simulink model "arm"  (R2018b)
settings: Solver=ode4  StartTime=0  StopTime=10  FixedStep=0.0005  RelTol=1e-7  AbsTol=1e-9  EnableMultiTasking=on
settings Model: Creator=Laksh  LastModifiedBy=visak
settings SolverCC: AutoScaleAbsTol=off  MaxConsecutiveMinStep=10  AlgebraicLoopSolver=LineSearch
settings DataIOCC: SaveFormat=StructureWithTime  SignalLogging=off  ReturnWorkspaceOutputs=on
settings OptimizationCC: LifeSpan=inf
settings DebuggingCC: ReadBeforeWriteMsg=DisableAll  WriteAfterWriteMsg=DisableAll  WriteAfterReadMsg=DisableAll  AlgebraicLoopMsg=none  MultiTaskDSMMsg=none  LibraryContextMissingDiagnostic=none  SFUnexpectedBacktrackingDiag=warning  SFNoUnconditionalDefaultTransitionDiag=warning  SFExecutionAtInitializationDiag=none
settings ModelReferenceCC: UpdateModelReferenceTargets=IfOutOfDate  ModelReferenceMinAlgLoopOccurrences=on
settings SFSimCC: SFSimEcho=off  SimUseLocalCustomCode=off
settings RTWCC: RTWUseLocalCustomCode=off
settings CodeAppCC: StateflowObjectComments=on
settings GRTTargetCC: TargetLangStandard=C89/C90 (ANSI)  GeneratePreprocessorConditionals=Disable all
settings ConfigComp: CovMetricSettings=dw  CovHtmlReporting=on  CovSaveCumulativeToWorkspaceVar=on  CovSaveSingleToWorkspaceVar=on  CovExternalEMLEnable=off

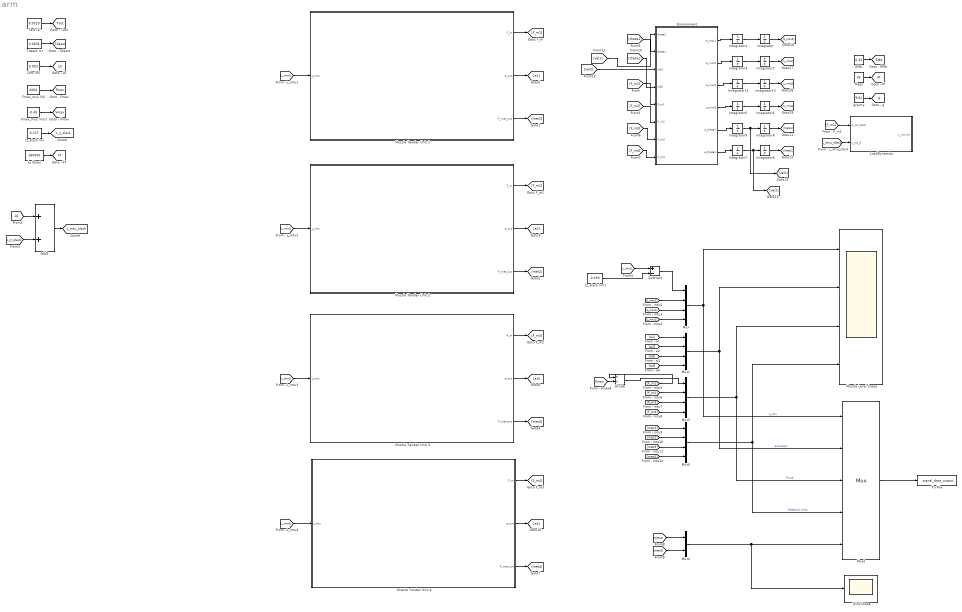
== system arm ==
  Add1 : Sum
  Divide : Product  Inputs=*/
  EMA : Constant  Value=0.33
  Environment : MATLAB Function  TreatAsAtomicUnit=on
  Fmax_mus (N) : Constant  Value=6000
  Integrator : Integrator  InitialCondition=0.05
  Integrator{1..11} (11 alike) : Integrator
  Joint Scope : Scope
  L0m (m) : Constant  Value=0.055
  LoadDynamics : Subsystem
  Lt_slack (m) : Constant  Value=0.237
  Lt_slack (m)1 : Constant  Value=0.293
  Mass : Constant  Value=35
  Muscle Level Scope : Scope  NumInputPorts=4
  Muscle Tenden Unit 1 : Subsystem
  Muscle Tenden Unit 2 : Subsystem
  Muscle Tenden Unit 3 : Subsystem
  Muscle Tenden Unit 4 : Subsystem
  Mux{,1,3,5} (4 alike) : Mux
  Mux2 : Mux  Inputs=5
      settings: DisplayOption=signals
  Mux4 : Mux  Inputs=2
  Subtract : Sum  Inputs=+-
  Tact (s) : Constant  Value=0.0329  VectorParams1D=off
  Tdeact (s) : Constant  Value=0.0905
  To File : ToFile  Filename=signal_data_output  MatrixName=data  SaveFormat=Timeseries
  Vmax_mus (m\s) : Constant  Value=-0.45
  gravity : Constant  Value=9.81
  kt (N\m) : Constant  Value=180000
  tag scope: EMA=global, Fmax=global, L0=global, L_mtu_slack=global, L_t_slack=global, M=global, Tact=global, Tdeact=global, Vmax=global, g=global, kT=global
  wires:
  Mux2/1 -> To File/1
  Tact (s)/1 -> [Tact]
  Tdeact (s)/1 -> [Tdeact]
  L0m (m)/1 -> [L0]
  Fmax_mus (N)/1 -> [Fmax]
  Vmax_mus (m\s)/1 -> [Vmax]
  Lt_slack (m)/1 -> [L_t_slack]
  [L_t_slack] -> Add1/2
  Add1/1 -> [L_mtu_slack]
  [L0] -> Add1/1
  kt (N\m)/1 -> [kT]
  [a1] -> Mux1/1
  [a2] -> Mux1/2
  Mux1/1 -> Muscle Level Scope/2, Mux2/2  "activation"
  Muscle Tenden Unit 1/1(F_m) -> [F_m1]
  [L_mtu1] -> Muscle Tenden Unit 1/1("L_mtu ")
  Muscle Tenden Unit 1/2(a_out) -> [a1]
  [F_m1] -> Environment/5(F_m1)
  [F_m2] -> Environment/6(F_m2)
  [F_m3] -> Environment/7(F_m3)
  [F_m4] -> Environment/8(F_m4)
  Environment/2(a_mtu2) -> Integrator3/1
  Muscle Tenden Unit 1/3(P_met_out) -> [met1]
  Muscle Tenden Unit 2/2(a_out) -> [a2]
  [L_mtu2] -> Muscle Tenden Unit 2/1("L_mtu ")
  Muscle Tenden Unit 2/1(F_m) -> [F_m2]
  Muscle Tenden Unit 2/3(P_met_out) -> [met2]
  Muscle Tenden Unit 3/3(P_met_out) -> [met3]
  Muscle Tenden Unit 3/1(F_m) -> [F_m3]
  [L_mtu3] -> Muscle Tenden Unit 3/1("L_mtu ")
  Muscle Tenden Unit 3/2(a_out) -> [a3]
  Muscle Tenden Unit 4/2(a_out) -> [a4]
  [L_mtu4] -> Muscle Tenden Unit 4/1("L_mtu ")
  Muscle Tenden Unit 4/1(F_m) -> [F_m4]
  Muscle Tenden Unit 4/3(P_met_out) -> [met4]
  [theta1] -> Mux4/1
  [theta2] -> Mux4/2
  [a3] -> Mux1/3
  [a4] -> Mux1/4
  [L_mtu1] -> Mux/3
  [L_mtu1] -> Mux/2
  [L_mtu1] -> Mux/4
  [F_m4] -> Mux3/4
  [F_m1] -> Divide/1
  [F_m3] -> Mux3/3
  [F_m2] -> Mux3/2
  Mux3/1 -> Muscle Level Scope/3, Mux2/3  "Force"
  Mux4/1 -> Mux2/5, Joint Scope/1
  Mux5/1 -> Muscle Level Scope/4, Mux2/4  "Metabolic Cost"
  [met2] -> Mux5/2
  [met3] -> Mux5/3
  [met1] -> Mux5/1
  [met4] -> Mux5/4
  Mux/1 -> Mux2/1, Muscle Level Scope/1  "L_mtu"
  Environment/1(a_mtu1) -> Integrator1/1
  Integrator1/1 -> Integrator/1
  Integrator3/1 -> Integrator2/1
  Integrator2/1 -> [L_mtu2]
  Integrator5/1 -> Integrator4/1
  Environment/4(a_mtu4) -> Integrator5/1
  Environment/6(a_theta2) -> Integrator7/1
  Integrator7/1 -> [vel2], Integrator6/1
  Integrator6/1 -> [theta2]
  Integrator4/1 -> [L_mtu4]
  Integrator8/1 -> [theta1]
  Integrator9/1 -> [vel1], Integrator8/1
  Environment/5(a_theta1) -> Integrator9/1
  Integrator11/1 -> Integrator10/1
  Environment/3(a_mtu3) -> Integrator11/1
  Integrator10/1 -> [L_mtu3]
  Integrator/1 -> [L_mtu1]
  [Fmax] -> Divide/2
  Divide/1 -> Mux3/1
  [L_mtu_slack] -> LoadDynamics/2(L_mt_0)
  [F_m1] -> LoadDynamics/1(F_mt_total)
  Mass/1 -> [M]
  gravity/1 -> [g]
  EMA/1 -> [EMA]
  Lt_slack (m)1/1 -> Subtract/2
  Subtract/1 -> Mux/1
  [L_mtu1] -> Subtract/1
  [theta2] -> Environment/3(vel1)
  [vel2] -> Environment/4(vel2)
  [vel1] -> Environment/1(theta2)
  [theta1] -> Environment/2(theta1)

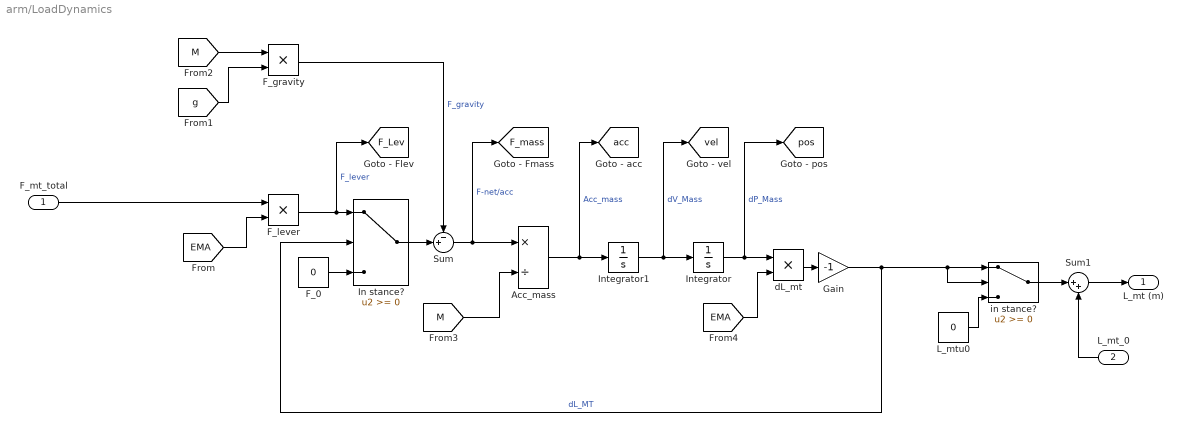
== system arm/LoadDynamics ==
  F_mt_total : Inport
  L_mt_0 : Inport  Port=2
  Acc_mass : Product  Inputs=*/
  F_0 : Constant  Value=0
  F_gravity : Product  RndMeth=Zero
  F_lever : Product  RndMeth=Zero
  Gain : Gain  Gain=-1
  In stance? : Switch
  Integrator : Integrator  InitialCondition=0.05
  Integrator1 : Integrator
  L_mtu0 : Constant  Value=0
  Sum : Sum  Inputs=-+|
  Sum1 : Sum  Inputs=|++
  dL_mt : Product  RndMeth=Zero
  "in stance? " : Switch
  L_mt (m) : Outport
  tag scope: F_Lev=global, F_mass=global, acc=global, pos=global, vel=global
  wires:
  Integrator1/1 -> [vel], Integrator/1  "dV_Mass"
  Sum1/1 -> L_mt (m)/1
  L_mt_0/1 -> Sum1/2
  Acc_mass/1 -> [acc], Integrator1/1  "Acc_mass"
  Sum/1 -> [F_mass], Acc_mass/1  "F-net/acc"
  F_mt_total/1 -> F_lever/1
  Gain/1 -> "in stance? "/2, "in stance? "/1, In stance?/2  "dL_MT"
  dL_mt/1 -> Gain/1
  F_lever/1 -> [F_Lev], In stance?/1  "F_lever"
  L_mtu0/1 -> "in stance? "/3
  "in stance? "/1 -> Sum1/1
  [M] -> F_gravity/1
  [g] -> F_gravity/2
  [EMA] -> F_lever/2
  F_0/1 -> In stance?/3
  Integrator/1 -> [pos], dL_mt/1  "dP_Mass"
  [M] -> Acc_mass/2
  In stance?/1 -> Sum/2
  F_gravity/1 -> Sum/1  "F_gravity"
  [EMA] -> dL_mt/2

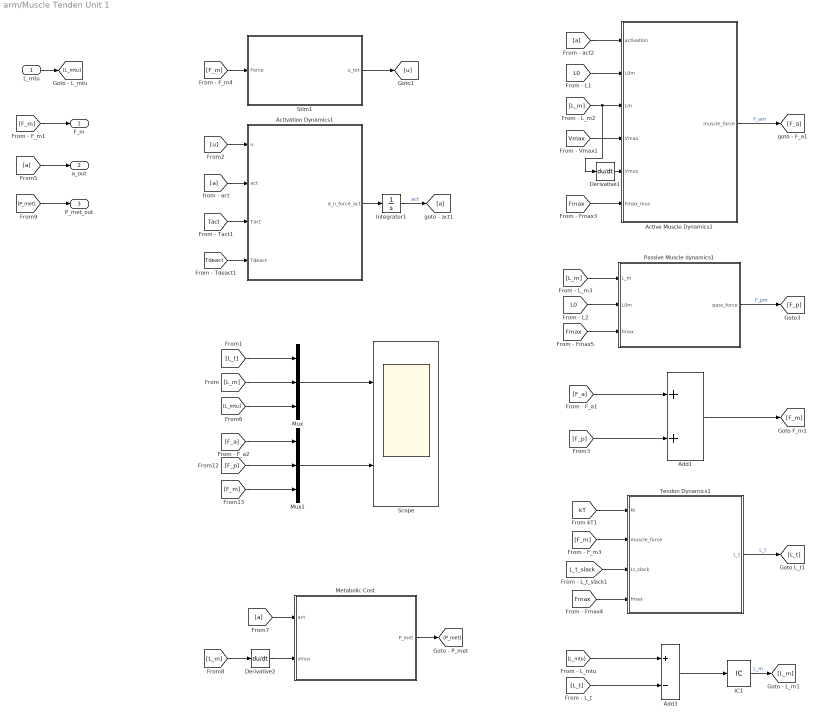
== system arm/Muscle Tenden Unit 1 ==
  "L_mtu " : Inport
  Activation Dynamics1 : MATLAB Function  TreatAsAtomicUnit=on
  Active Muscle Dynamics1 : MATLAB Function
  Add1 : Sum
  Add3 : Sum  Inputs=+-
  Derivative1 : Derivative
  Derivative2 : Derivative
  IC1 : InitialCondition  Value=0.05
  Integrator1 : Integrator
  Metabolic Cost : MATLAB Function
  Mux : Mux  Inputs=3
  Mux1 : Mux  Inputs=3
  Passive Muscle dynamics1 : MATLAB Function
  Scope : Scope  NumInputPorts=2
  Stim1 : Subsystem
  Tendon Dynamics1 : MATLAB Function
  F_m : Outport
  a_out : Outport  Port=2
  P_met_out : Outport  Port=3
  wires:
  [F_m] -> F_m/1
  Activation Dynamics1/1(d_n_force_act) -> Integrator1/1
  [F_p] -> Add1/2
  [L_m] -> Passive Muscle dynamics1/1(L_m)
  [L_mtu] -> Add3/1
  [L_m] -> Derivative1/1, Active Muscle Dynamics1/3(Lm)
  Stim1/1(u_tot) -> [u]
  [F_m] -> Stim1/1(Force)
  Tendon Dynamics1/1(L_t) -> [L_t]  "L_t"
  Add1/1 -> [F_m]
  [a] -> Active Muscle Dynamics1/1(activation)
  Passive Muscle dynamics1/1(pass_force) -> [F_p]  "F_pm"
  [Fmax] -> Passive Muscle dynamics1/3(fmax)
  [kT] -> Tendon Dynamics1/1(kt)
  [L_t] -> Add3/2
  [Vmax] -> Active Muscle Dynamics1/4(Vmax)
  [Fmax] -> Tendon Dynamics1/4(fmax)
  [L0] -> Passive Muscle dynamics1/2(L0m)
  [L_t_slack] -> Tendon Dynamics1/3(Lt_slack)
  [Fmax] -> Active Muscle Dynamics1/6(Fmax_mus)
  [Tact] -> Activation Dynamics1/3(Tact)
  [L0] -> Active Muscle Dynamics1/2(L0m)
  IC1/1 -> [L_m]  "L_m"
  [u] -> Activation Dynamics1/1(u)
  Integrator1/1 -> [a]  "act"
  [F_a] -> Add1/1
  [Tdeact] -> Activation Dynamics1/4(Tdeact)
  Derivative1/1 -> Active Muscle Dynamics1/5(Vmus)
  [a] -> Activation Dynamics1/2(act)
  [F_m] -> Tendon Dynamics1/2(muscle_force)
  Active Muscle Dynamics1/1(muscle_force) -> [F_a]  "F_am"
  Add3/1 -> IC1/1
  "L_mtu "/1 -> [L_mtu]
  [L_m] -> Mux/2
  [L_t] -> Mux/1
  [a] -> a_out/1
  [a] -> Metabolic Cost/1(act)
  [L_m] -> Derivative2/1
  Derivative2/1 -> Metabolic Cost/2(vmus)
  Metabolic Cost/1(P_met) -> [P_met]
  [P_met] -> P_met_out/1
  [L_mtu] -> Mux/3
  Mux/1 -> Scope/1
  [F_a] -> Mux1/1
  [F_m] -> Mux1/3
  [F_p] -> Mux1/2
  Mux1/1 -> Scope/2

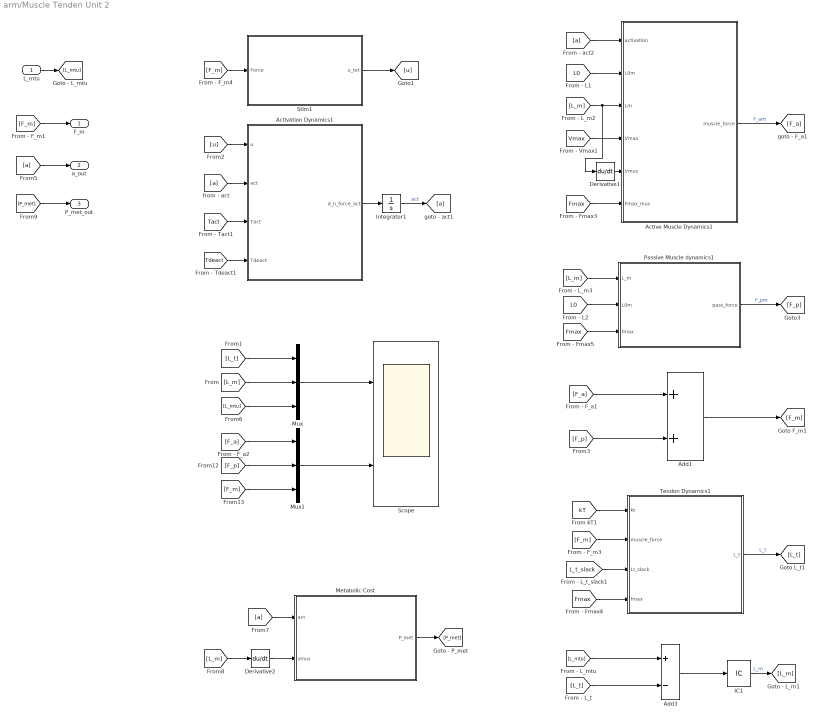
== system arm/Muscle Tenden Unit 2 ==
  "L_mtu " : Inport
  Activation Dynamics1 : MATLAB Function  TreatAsAtomicUnit=on
  Active Muscle Dynamics1 : MATLAB Function
  Add1 : Sum
  Add3 : Sum  Inputs=+-
  Derivative1 : Derivative
  Derivative2 : Derivative
  IC1 : InitialCondition  Value=0.05
  Integrator1 : Integrator
  Metabolic Cost : MATLAB Function
  Mux : Mux  Inputs=3
  Mux1 : Mux  Inputs=3
  Passive Muscle dynamics1 : MATLAB Function
  Scope : Scope  NumInputPorts=2
  Stim1 : Subsystem
  Tendon Dynamics1 : MATLAB Function
  F_m : Outport
  a_out : Outport  Port=2
  P_met_out : Outport  Port=3
  wires:
  [F_m] -> F_m/1
  Activation Dynamics1/1(d_n_force_act) -> Integrator1/1
  [F_p] -> Add1/2
  [L_m] -> Passive Muscle dynamics1/1(L_m)
  [L_mtu] -> Add3/1
  [L_m] -> Derivative1/1, Active Muscle Dynamics1/3(Lm)
  Stim1/1(u_tot) -> [u]
  [F_m] -> Stim1/1(Force)
  Tendon Dynamics1/1(L_t) -> [L_t]  "L_t"
  Add1/1 -> [F_m]
  [a] -> Active Muscle Dynamics1/1(activation)
  Passive Muscle dynamics1/1(pass_force) -> [F_p]  "F_pm"
  [Fmax] -> Passive Muscle dynamics1/3(fmax)
  [kT] -> Tendon Dynamics1/1(kt)
  [L_t] -> Add3/2
  [Vmax] -> Active Muscle Dynamics1/4(Vmax)
  [Fmax] -> Tendon Dynamics1/4(fmax)
  [L0] -> Passive Muscle dynamics1/2(L0m)
  [L_t_slack] -> Tendon Dynamics1/3(Lt_slack)
  [Fmax] -> Active Muscle Dynamics1/6(Fmax_mus)
  [Tact] -> Activation Dynamics1/3(Tact)
  [L0] -> Active Muscle Dynamics1/2(L0m)
  IC1/1 -> [L_m]  "L_m"
  [u] -> Activation Dynamics1/1(u)
  Integrator1/1 -> [a]  "act"
  [F_a] -> Add1/1
  [Tdeact] -> Activation Dynamics1/4(Tdeact)
  Derivative1/1 -> Active Muscle Dynamics1/5(Vmus)
  [a] -> Activation Dynamics1/2(act)
  [F_m] -> Tendon Dynamics1/2(muscle_force)
  Active Muscle Dynamics1/1(muscle_force) -> [F_a]  "F_am"
  Add3/1 -> IC1/1
  "L_mtu "/1 -> [L_mtu]
  [L_m] -> Mux/2
  [L_t] -> Mux/1
  [a] -> a_out/1
  [a] -> Metabolic Cost/1(act)
  [L_m] -> Derivative2/1
  Derivative2/1 -> Metabolic Cost/2(vmus)
  Metabolic Cost/1(P_met) -> [P_met]
  [P_met] -> P_met_out/1
  [L_mtu] -> Mux/3
  Mux/1 -> Scope/1
  [F_a] -> Mux1/1
  [F_m] -> Mux1/3
  [F_p] -> Mux1/2
  Mux1/1 -> Scope/2

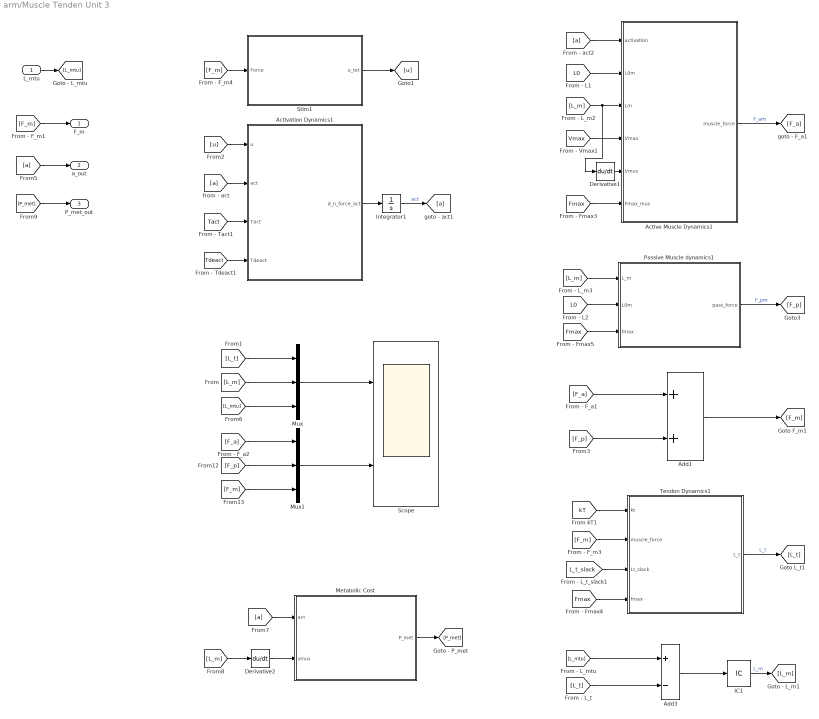
== system arm/Muscle Tenden Unit 3 ==
  "L_mtu " : Inport
  Activation Dynamics1 : MATLAB Function  TreatAsAtomicUnit=on
  Active Muscle Dynamics1 : MATLAB Function
  Add1 : Sum
  Add3 : Sum  Inputs=+-
  Derivative1 : Derivative
  Derivative2 : Derivative
  IC1 : InitialCondition  Value=0.05
  Integrator1 : Integrator
  Metabolic Cost : MATLAB Function
  Mux : Mux  Inputs=3
  Mux1 : Mux  Inputs=3
  Passive Muscle dynamics1 : MATLAB Function
  Scope : Scope  NumInputPorts=2
  Stim1 : Subsystem
  Tendon Dynamics1 : MATLAB Function
  F_m : Outport
  a_out : Outport  Port=2
  P_met_out : Outport  Port=3
  wires:
  [F_m] -> F_m/1
  Activation Dynamics1/1(d_n_force_act) -> Integrator1/1
  [F_p] -> Add1/2
  [L_m] -> Passive Muscle dynamics1/1(L_m)
  [L_mtu] -> Add3/1
  [L_m] -> Derivative1/1, Active Muscle Dynamics1/3(Lm)
  Stim1/1(u_tot) -> [u]
  [F_m] -> Stim1/1(Force)
  Tendon Dynamics1/1(L_t) -> [L_t]  "L_t"
  Add1/1 -> [F_m]
  [a] -> Active Muscle Dynamics1/1(activation)
  Passive Muscle dynamics1/1(pass_force) -> [F_p]  "F_pm"
  [Fmax] -> Passive Muscle dynamics1/3(fmax)
  [kT] -> Tendon Dynamics1/1(kt)
  [L_t] -> Add3/2
  [Vmax] -> Active Muscle Dynamics1/4(Vmax)
  [Fmax] -> Tendon Dynamics1/4(fmax)
  [L0] -> Passive Muscle dynamics1/2(L0m)
  [L_t_slack] -> Tendon Dynamics1/3(Lt_slack)
  [Fmax] -> Active Muscle Dynamics1/6(Fmax_mus)
  [Tact] -> Activation Dynamics1/3(Tact)
  [L0] -> Active Muscle Dynamics1/2(L0m)
  IC1/1 -> [L_m]  "L_m"
  [u] -> Activation Dynamics1/1(u)
  Integrator1/1 -> [a]  "act"
  [F_a] -> Add1/1
  [Tdeact] -> Activation Dynamics1/4(Tdeact)
  Derivative1/1 -> Active Muscle Dynamics1/5(Vmus)
  [a] -> Activation Dynamics1/2(act)
  [F_m] -> Tendon Dynamics1/2(muscle_force)
  Active Muscle Dynamics1/1(muscle_force) -> [F_a]  "F_am"
  Add3/1 -> IC1/1
  "L_mtu "/1 -> [L_mtu]
  [L_m] -> Mux/2
  [L_t] -> Mux/1
  [a] -> a_out/1
  [a] -> Metabolic Cost/1(act)
  [L_m] -> Derivative2/1
  Derivative2/1 -> Metabolic Cost/2(vmus)
  Metabolic Cost/1(P_met) -> [P_met]
  [P_met] -> P_met_out/1
  [L_mtu] -> Mux/3
  Mux/1 -> Scope/1
  [F_a] -> Mux1/1
  [F_m] -> Mux1/3
  [F_p] -> Mux1/2
  Mux1/1 -> Scope/2

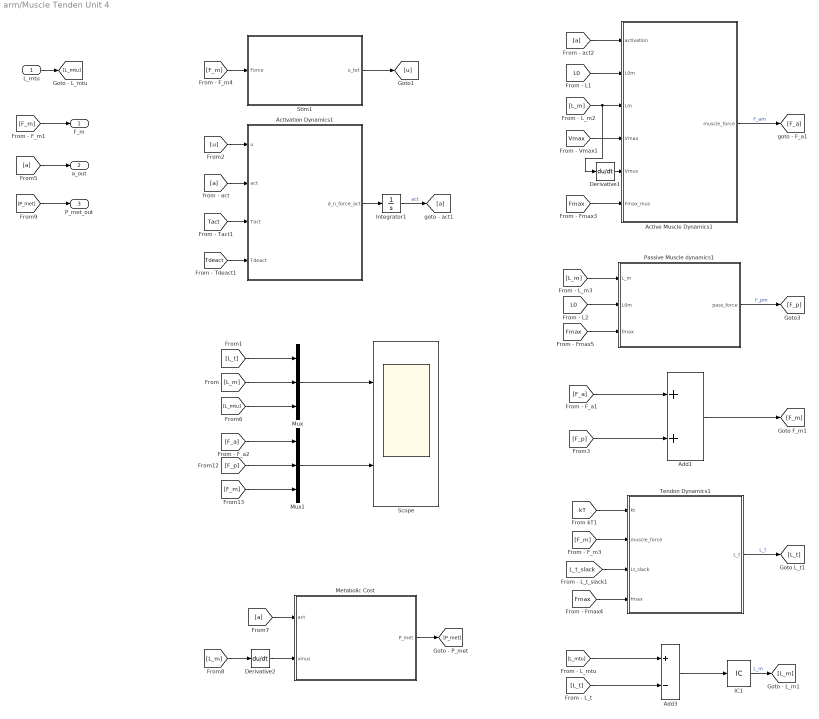
== system arm/Muscle Tenden Unit 4 ==
  "L_mtu " : Inport
  Activation Dynamics1 : MATLAB Function  TreatAsAtomicUnit=on
  Active Muscle Dynamics1 : MATLAB Function
  Add1 : Sum
  Add3 : Sum  Inputs=+-
  Derivative1 : Derivative
  Derivative2 : Derivative
  IC1 : InitialCondition  Value=0.05
  Integrator1 : Integrator
  Metabolic Cost : MATLAB Function
  Mux : Mux  Inputs=3
  Mux1 : Mux  Inputs=3
  Passive Muscle dynamics1 : MATLAB Function
  Scope : Scope  NumInputPorts=2
  Stim1 : Subsystem
  Tendon Dynamics1 : MATLAB Function
  F_m : Outport
  a_out : Outport  Port=2
  P_met_out : Outport  Port=3
  wires:
  [F_m] -> F_m/1
  Activation Dynamics1/1(d_n_force_act) -> Integrator1/1
  [F_p] -> Add1/2
  [L_m] -> Passive Muscle dynamics1/1(L_m)
  [L_mtu] -> Add3/1
  [L_m] -> Derivative1/1, Active Muscle Dynamics1/3(Lm)
  Stim1/1(u_tot) -> [u]
  [F_m] -> Stim1/1(Force)
  Tendon Dynamics1/1(L_t) -> [L_t]  "L_t"
  Add1/1 -> [F_m]
  [a] -> Active Muscle Dynamics1/1(activation)
  Passive Muscle dynamics1/1(pass_force) -> [F_p]  "F_pm"
  [Fmax] -> Passive Muscle dynamics1/3(fmax)
  [kT] -> Tendon Dynamics1/1(kt)
  [L_t] -> Add3/2
  [Vmax] -> Active Muscle Dynamics1/4(Vmax)
  [Fmax] -> Tendon Dynamics1/4(fmax)
  [L0] -> Passive Muscle dynamics1/2(L0m)
  [L_t_slack] -> Tendon Dynamics1/3(Lt_slack)
  [Fmax] -> Active Muscle Dynamics1/6(Fmax_mus)
  [Tact] -> Activation Dynamics1/3(Tact)
  [L0] -> Active Muscle Dynamics1/2(L0m)
  IC1/1 -> [L_m]  "L_m"
  [u] -> Activation Dynamics1/1(u)
  Integrator1/1 -> [a]  "act"
  [F_a] -> Add1/1
  [Tdeact] -> Activation Dynamics1/4(Tdeact)
  Derivative1/1 -> Active Muscle Dynamics1/5(Vmus)
  [a] -> Activation Dynamics1/2(act)
  [F_m] -> Tendon Dynamics1/2(muscle_force)
  Active Muscle Dynamics1/1(muscle_force) -> [F_a]  "F_am"
  Add3/1 -> IC1/1
  "L_mtu "/1 -> [L_mtu]
  [L_m] -> Mux/2
  [L_t] -> Mux/1
  [a] -> a_out/1
  [a] -> Metabolic Cost/1(act)
  [L_m] -> Derivative2/1
  Derivative2/1 -> Metabolic Cost/2(vmus)
  Metabolic Cost/1(P_met) -> [P_met]
  [P_met] -> P_met_out/1
  [L_mtu] -> Mux/3
  Mux/1 -> Scope/1
  [F_a] -> Mux1/1
  [F_m] -> Mux1/3
  [F_p] -> Mux1/2
  Mux1/1 -> Scope/2

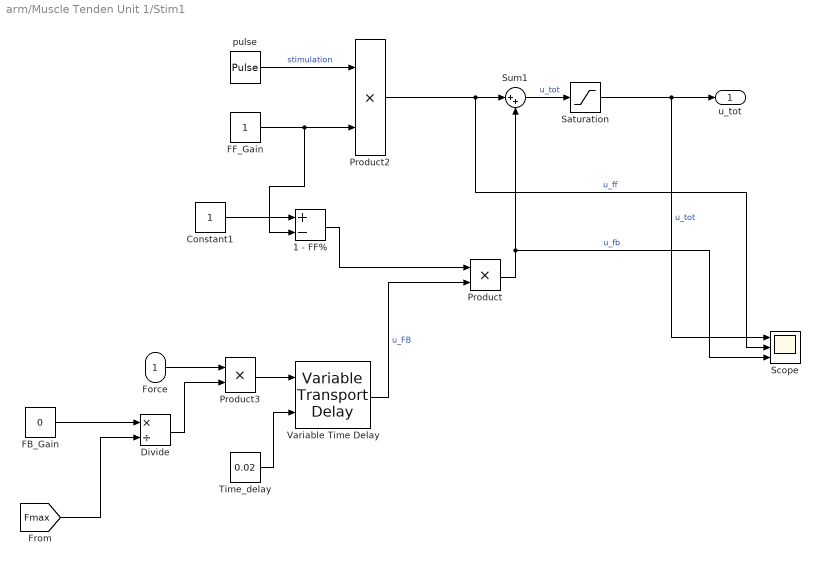
== system arm/Muscle Tenden Unit 1/Stim1 ==
  Force : Inport
  1 - FF% : Sum  Inputs=+-
  Constant1 : Constant
  Divide : Product  Inputs=*/
  FB_Gain : Constant  Value=0
  FF_Gain : Constant
  Product : Product
  Product2 : Product
  Product3 : Product
  Saturation : Saturate  UpperLimit=1  LowerLimit=0
  Scope : Scope  NumInputPorts=3
  Sum1 : Sum  Inputs=|++
  Time_delay : Constant  Value=0.02
  Variable Time Delay : VariableTransportDelay  MaximumDelay=10  MaximumPoints=40960
  pulse : DiscretePulseGenerator  PulseType=Time based  Period=0.4  PulseWidth=10  PhaseDelay=0.1
  u_tot : Outport
  wires:
  pulse/1 -> Product2/1  "stimulation"
  FF_Gain/1 -> 1 - FF%/2, Product2/2
  Variable Time Delay/1 -> Product/2  "u_FB"
  Time_delay/1 -> Variable Time Delay/2
  Product3/1 -> Variable Time Delay/1
  Constant1/1 -> 1 - FF%/1
  Sum1/1 -> Saturation/1  "u_tot"
  1 - FF%/1 -> Product/1
  Product2/1 -> Scope/2, Sum1/1  "u_ff"
  Product/1 -> Scope/3, Sum1/2  "u_fb"
  Saturation/1 -> Scope/1, u_tot/1  "u_tot"
  FB_Gain/1 -> Divide/1
  [Fmax] -> Divide/2
  Divide/1 -> Product3/2
  Force/1 -> Product3/1

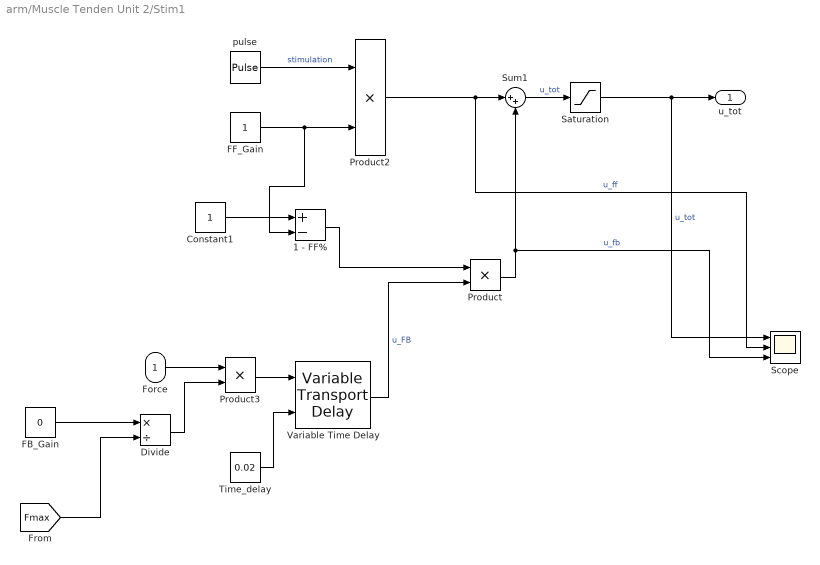
== system arm/Muscle Tenden Unit 2/Stim1 ==
  Force : Inport
  1 - FF% : Sum  Inputs=+-
  Constant1 : Constant
  Divide : Product  Inputs=*/
  FB_Gain : Constant  Value=0
  FF_Gain : Constant
  Product : Product
  Product2 : Product
  Product3 : Product
  Saturation : Saturate  UpperLimit=1  LowerLimit=0
  Scope : Scope  NumInputPorts=3
  Sum1 : Sum  Inputs=|++
  Time_delay : Constant  Value=0.02
  Variable Time Delay : VariableTransportDelay  MaximumDelay=10  MaximumPoints=40960
  pulse : DiscretePulseGenerator  PulseType=Time based  Period=0.4  PulseWidth=10  PhaseDelay=0.1
  u_tot : Outport
  wires:
  pulse/1 -> Product2/1  "stimulation"
  FF_Gain/1 -> 1 - FF%/2, Product2/2
  Variable Time Delay/1 -> Product/2  "u_FB"
  Time_delay/1 -> Variable Time Delay/2
  Product3/1 -> Variable Time Delay/1
  Constant1/1 -> 1 - FF%/1
  Sum1/1 -> Saturation/1  "u_tot"
  1 - FF%/1 -> Product/1
  Product2/1 -> Scope/2, Sum1/1  "u_ff"
  Product/1 -> Scope/3, Sum1/2  "u_fb"
  Saturation/1 -> Scope/1, u_tot/1  "u_tot"
  FB_Gain/1 -> Divide/1
  [Fmax] -> Divide/2
  Divide/1 -> Product3/2
  Force/1 -> Product3/1

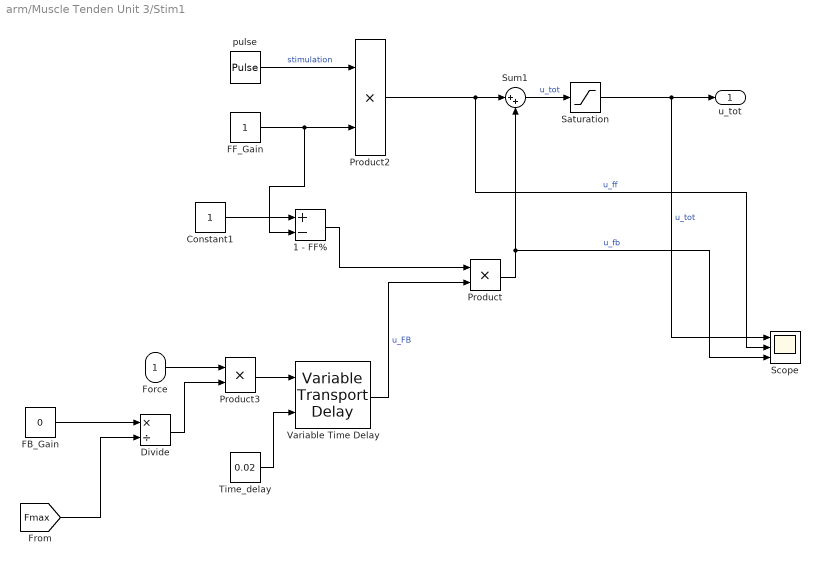
== system arm/Muscle Tenden Unit 3/Stim1 ==
  Force : Inport
  1 - FF% : Sum  Inputs=+-
  Constant1 : Constant
  Divide : Product  Inputs=*/
  FB_Gain : Constant  Value=0
  FF_Gain : Constant
  Product : Product
  Product2 : Product
  Product3 : Product
  Saturation : Saturate  UpperLimit=1  LowerLimit=0
  Scope : Scope  NumInputPorts=3
  Sum1 : Sum  Inputs=|++
  Time_delay : Constant  Value=0.02
  Variable Time Delay : VariableTransportDelay  MaximumDelay=10  MaximumPoints=40960
  pulse : DiscretePulseGenerator  PulseType=Time based  Period=0.4  PulseWidth=10  PhaseDelay=0.1
  u_tot : Outport
  wires:
  pulse/1 -> Product2/1  "stimulation"
  FF_Gain/1 -> 1 - FF%/2, Product2/2
  Variable Time Delay/1 -> Product/2  "u_FB"
  Time_delay/1 -> Variable Time Delay/2
  Product3/1 -> Variable Time Delay/1
  Constant1/1 -> 1 - FF%/1
  Sum1/1 -> Saturation/1  "u_tot"
  1 - FF%/1 -> Product/1
  Product2/1 -> Scope/2, Sum1/1  "u_ff"
  Product/1 -> Scope/3, Sum1/2  "u_fb"
  Saturation/1 -> Scope/1, u_tot/1  "u_tot"
  FB_Gain/1 -> Divide/1
  [Fmax] -> Divide/2
  Divide/1 -> Product3/2
  Force/1 -> Product3/1

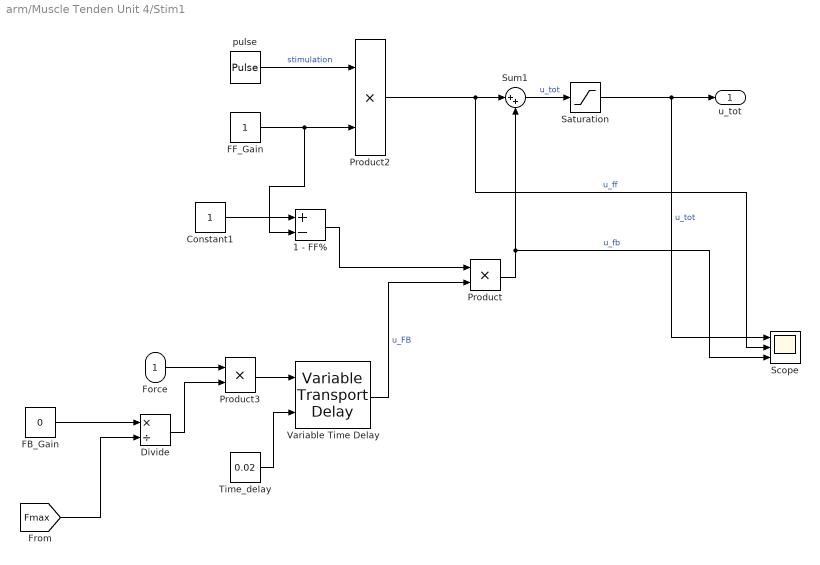
== system arm/Muscle Tenden Unit 4/Stim1 ==
  Force : Inport
  1 - FF% : Sum  Inputs=+-
  Constant1 : Constant
  Divide : Product  Inputs=*/
  FB_Gain : Constant  Value=0
  FF_Gain : Constant
  Product : Product
  Product2 : Product
  Product3 : Product
  Saturation : Saturate  UpperLimit=1  LowerLimit=0
  Scope : Scope  NumInputPorts=3
  Sum1 : Sum  Inputs=|++
  Time_delay : Constant  Value=0.02
  Variable Time Delay : VariableTransportDelay  MaximumDelay=10  MaximumPoints=40960
  pulse : DiscretePulseGenerator  PulseType=Time based  Period=0.4  PulseWidth=10  PhaseDelay=0.1
  u_tot : Outport
  wires:
  pulse/1 -> Product2/1  "stimulation"
  FF_Gain/1 -> 1 - FF%/2, Product2/2
  Variable Time Delay/1 -> Product/2  "u_FB"
  Time_delay/1 -> Variable Time Delay/2
  Product3/1 -> Variable Time Delay/1
  Constant1/1 -> 1 - FF%/1
  Sum1/1 -> Saturation/1  "u_tot"
  1 - FF%/1 -> Product/1
  Product2/1 -> Scope/2, Sum1/1  "u_ff"
  Product/1 -> Scope/3, Sum1/2  "u_fb"
  Saturation/1 -> Scope/1, u_tot/1  "u_tot"
  FB_Gain/1 -> Divide/1
  [Fmax] -> Divide/2
  Divide/1 -> Product3/2
  Force/1 -> Product3/1

== matlab function arm/Muscle Tenden Unit 3/Activation Dynamics1 ==
  data: u input; d_n_force_act output; act input; Tact input; Tdeact input
function d_n_force_act = d_n_force_act(u,act,Tact,Tdeact)
%#codegen    
%Rate of change of activation
%Equation is taken from Zajac (1989) Eq. 1
    B=Tact/Tdeact;
    d_n_force_act= u/Tact - (1/Tact*(B+(1-B)*u))*act;
end

== matlab function arm/Muscle Tenden Unit 3/Active Muscle Dynamics1 ==
  data: activation input; L0m input; Lm input; Vmax input; Vmus input; Fmax_mus input; muscle_force output
function muscle_force   =...
    muscle_dynamics(activation,L0m,Lm,Vmax,Vmus,Fmax_mus)
%#codegen

    %Hill Type Muscle F-V relationship.  Returns a normalized force-velocity value
    if (Vmus<Vmax)
        n_force_velocity=0;
    else
        if (Vmus >= Vmax && Vmus < 0)
            n_force_velocity = ((1-(Vmus/Vmax))/(1+(Vmus/0.17/Vmax)));
        else
            n_force_velocity =(1.8-0.8*((1+(Vmus/Vmax))/(1-7.56*Vmus/0.17/Vmax)));
        end
    end
    
    %Active muscle F-L relationships.  Returns a normalized F-L value

    a = 3.1108;
    b = .8698;
    s = .3914;

    if Lm < 0
        Lm = 0;
    end

    n_force_length = exp(-(abs(((Lm/L0m)^b-1)/s))^a);

    %Total active force of muscle based on normalized F-V and F-L relationships
    muscle_force = Fmax_mus* activation * n_force_velocity * n_force_length;
end

== matlab function arm/Muscle Tenden Unit 3/Metabolic Cost ==
  data: P_met output; act input; vmus input
function P_met = metabolic_cost(act, vmus)

    vmax = -0.45;
    Fmax = 6000;

    isLengthening = vmus > 0;
    isShortening = vmus <= 0; 

    psi = (0.01-(0.11*(vmus/vmax))+(0.06*exp(23*vmus/vmax))).*isLengthening;
    psi = psi + (0.23-0.16*exp(-8*vmus/vmax)).*isShortening;

    P_met = psi.*act.*abs(Fmax*vmax);

end

== matlab function arm/Muscle Tenden Unit 3/Passive Muscle dynamics1 ==
  data: pass_force output; L_m input; L0m input; fmax input
function pass_force = pmuscle_dynamics(L_m, L0m,fmax)
%#codegen
%passive CE F_L taken from Rubenson et. al.

%Passive muscle force
A = 2.38*10^(-2);
b = 5.31;

if L_m > 0    
    pass_force= fmax*A*exp(b*((L_m/L0m)-1));
else
    pass_force=0;
end


end

== matlab function arm/Environment ==
  data: theta2 input; theta1 input; vel1 input; vel2 input; F_m1 input; a_mtu1 output; a_mtu2 output; F_m2 input; F_m3 input; F_m4 input; a_mtu3 output; a_mtu4 output; a_theta1 output; a_theta2 output
function [a_mtu1,a_mtu2,a_mtu3,a_mtu4,a_theta1,a_theta2]  =...
    environment_response(theta2, theta1, vel1, vel2, F_m1,F_m2,F_m3,F_m4)
    m=35;
    EMA=0.33;
    x = [theta1,theta2,vel1,vel2];
    a_mtu1=-EMA*F_m1/m;
    a_mtu2=-F_m2/m-9.8;
    a_mtu3=-F_m3/m-9.8;
    a_mtu4=-F_m4/m-9.8;
    a_theta1=0;
    a_theta2=0;
    % Just a test, will have to update on the Joint-configuration dependent
    % moment arms
    moment_arm1 = 0.2;
    moment_arm2 = 0.2;
    moment_arm3 = 0.2;
    moment_arm4 = 0.2;

    %Torques
    net_Torque1 = F_m1*moment_arm1 - F_m2*moment_arm2;
    net_Torque2 = F_m3*moment_arm3 - F_m4*moment_arm4;
    F = [net_Torque1; net_Torque2];
    % Robot Specifications
    M1=1.0;
    M2=1.0;
    L1=1.0;
    L2=1.0;
    g=9.8;
    % Inertia Matrix
    b11=(M1+M2)*L1^2+M2*L2^2+2*M2*L1*L2*cos(x(2));
    b12=M2*L2^2+M2*L1*L2*cos(x(2));
    b21=M2*L2^2+M2*L1*L2*cos(x(2));
    b22=M2*L2^2;
    Bq=[b11 b12;b21 b22];
    % C Matrix
    c1=-M2*L1*L2*sin(x(2))*(2*x(3)*x(4)+x(4)^2);
    c2=-M2*L1*L2*sin(x(2))*x(3)*x(4);
    Cq=[c1;c2];
    % Gravity Matrix
    g1=-(M1+M2)*g*L1*sin(x(1))-M2*g*L2*sin(x(1)+x(2));
    g2=-M2*g*L2*sin(x(1)+x(2));
    Gq=[g1;g2];


    acceleration =inv(Bq)*(-Cq-Gq+F);
    
    a_theta1 = acceleration(1);
    a_theta2 = acceleration(2);
    

end

== matlab function arm/Muscle Tenden Unit 1/Activation Dynamics1 ==
  data: u input; d_n_force_act output; act input; Tact input; Tdeact input
function d_n_force_act = d_n_force_act(u,act,Tact,Tdeact)
%#codegen    
%Rate of change of activation
%Equation is taken from Zajac (1989) Eq. 1
    B=Tact/Tdeact;
    d_n_force_act= u/Tact - (1/Tact*(B+(1-B)*u))*act;
end

== matlab function arm/Muscle Tenden Unit 1/Active Muscle Dynamics1 ==
  data: activation input; L0m input; Lm input; Vmax input; Vmus input; Fmax_mus input; muscle_force output
function muscle_force   =...
    muscle_dynamics(activation,L0m,Lm,Vmax,Vmus,Fmax_mus)
%#codegen

    %Hill Type Muscle F-V relationship.  Returns a normalized force-velocity value
    if (Vmus<Vmax)
        n_force_velocity=0;
    else
        if (Vmus >= Vmax && Vmus < 0)
            n_force_velocity = ((1-(Vmus/Vmax))/(1+(Vmus/0.17/Vmax)));
        else
            n_force_velocity =(1.8-0.8*((1+(Vmus/Vmax))/(1-7.56*Vmus/0.17/Vmax)));
        end
    end
    
    %Active muscle F-L relationships.  Returns a normalized F-L value

    a = 3.1108;
    b = .8698;
    s = .3914;

    if Lm < 0
        Lm = 0;
    end

    n_force_length = exp(-(abs(((Lm/L0m)^b-1)/s))^a);

    %Total active force of muscle based on normalized F-V and F-L relationships
    muscle_force = Fmax_mus* activation * n_force_velocity * n_force_length;
end

== matlab function arm/Muscle Tenden Unit 1/Passive Muscle dynamics1 ==
  data: pass_force output; L_m input; L0m input; fmax input
function pass_force = pmuscle_dynamics(L_m, L0m,fmax)
%#codegen
%passive CE F_L taken from Rubenson et. al.

%Passive muscle force
A = 2.38*10^(-2);
b = 5.31;

if L_m > 0    
    pass_force= fmax*A*exp(b*((L_m/L0m)-1));
else
    pass_force=0;
end


end

== matlab function arm/Muscle Tenden Unit 1/Tendon Dynamics1 ==
  data: kt input; L_t output; muscle_force input; Lt_slack input; fmax input
function L_t = L_tendon(kt,muscle_force,Lt_slack,fmax)
%#codegen
%Lichtwark, G.A. and Wilson, A.M., 2008. Journal of theoretical biology, 252(4), pp.662-673.
%Total tendon length
dL_t = (muscle_force + (fmax*log((-9*exp(-(20*muscle_force)/fmax)) + 10))/20)/kt;
L_t = dL_t + Lt_slack ;

end

== matlab function arm/Muscle Tenden Unit 3/Tendon Dynamics1 ==
  data: kt input; L_t output; muscle_force input; Lt_slack input; fmax input
function L_t = L_tendon(kt,muscle_force,Lt_slack,fmax)
%#codegen
%Lichtwark, G.A. and Wilson, A.M., 2008. Journal of theoretical biology, 252(4), pp.662-673.
%Total tendon length
dL_t = (muscle_force + (fmax*log((-9*exp(-(20*muscle_force)/fmax)) + 10))/20)/kt;
L_t = dL_t + Lt_slack ;

end

== matlab function arm/Muscle Tenden Unit 4/Activation Dynamics1 ==
  data: u input; d_n_force_act output; act input; Tact input; Tdeact input
function d_n_force_act = d_n_force_act(u,act,Tact,Tdeact)
%#codegen    
%Rate of change of activation
%Equation is taken from Zajac (1989) Eq. 1
    B=Tact/Tdeact;
    d_n_force_act= u/Tact - (1/Tact*(B+(1-B)*u))*act;
end

== matlab function arm/Muscle Tenden Unit 4/Active Muscle Dynamics1 ==
  data: activation input; L0m input; Lm input; Vmax input; Vmus input; Fmax_mus input; muscle_force output
function muscle_force   =...
    muscle_dynamics(activation,L0m,Lm,Vmax,Vmus,Fmax_mus)
%#codegen

    %Hill Type Muscle F-V relationship.  Returns a normalized force-velocity value
    if (Vmus<Vmax)
        n_force_velocity=0;
    else
        if (Vmus >= Vmax && Vmus < 0)
            n_force_velocity = ((1-(Vmus/Vmax))/(1+(Vmus/0.17/Vmax)));
        else
            n_force_velocity =(1.8-0.8*((1+(Vmus/Vmax))/(1-7.56*Vmus/0.17/Vmax)));
        end
    end
    
    %Active muscle F-L relationships.  Returns a normalized F-L value

    a = 3.1108;
    b = .8698;
    s = .3914;

    if Lm < 0
        Lm = 0;
    end

    n_force_length = exp(-(abs(((Lm/L0m)^b-1)/s))^a);

    %Total active force of muscle based on normalized F-V and F-L relationships
    muscle_force = Fmax_mus* activation * n_force_velocity * n_force_length;
end

== matlab function arm/Muscle Tenden Unit 4/Metabolic Cost ==
  data: P_met output; act input; vmus input
function P_met = metabolic_cost(act, vmus)

    vmax = -0.45;
    Fmax = 6000;

    isLengthening = vmus > 0;
    isShortening = vmus <= 0; 

    psi = (0.01-(0.11*(vmus/vmax))+(0.06*exp(23*vmus/vmax))).*isLengthening;
    psi = psi + (0.23-0.16*exp(-8*vmus/vmax)).*isShortening;

    P_met = psi.*act.*abs(Fmax*vmax);

end

== matlab function arm/Muscle Tenden Unit 4/Passive Muscle dynamics1 ==
  data: pass_force output; L_m input; L0m input; fmax input
function pass_force = pmuscle_dynamics(L_m, L0m,fmax)
%#codegen
%passive CE F_L taken from Rubenson et. al.

%Passive muscle force
A = 2.38*10^(-2);
b = 5.31;

if L_m > 0    
    pass_force= fmax*A*exp(b*((L_m/L0m)-1));
else
    pass_force=0;
end


end

== matlab function arm/Muscle Tenden Unit 4/Tendon Dynamics1 ==
  data: kt input; L_t output; muscle_force input; Lt_slack input; fmax input
function L_t = L_tendon(kt,muscle_force,Lt_slack,fmax)
%#codegen
%Lichtwark, G.A. and Wilson, A.M., 2008. Journal of theoretical biology, 252(4), pp.662-673.
%Total tendon length
dL_t = (muscle_force + (fmax*log((-9*exp(-(20*muscle_force)/fmax)) + 10))/20)/kt;
L_t = dL_t + Lt_slack ;

end

== matlab function arm/Muscle Tenden Unit 1/Metabolic Cost ==
  data: P_met output; act input; vmus input
function P_met = metabolic_cost(act, vmus)

    vmax = -0.45;
    Fmax = 6000;

    isLengthening = vmus > 0;
    isShortening = vmus <= 0; 

    psi = (0.01-(0.11*(vmus/vmax))+(0.06*exp(23*vmus/vmax))).*isLengthening;
    psi = psi + (0.23-0.16*exp(-8*vmus/vmax)).*isShortening;

    P_met = psi.*act.*abs(Fmax*vmax);

end

== matlab function arm/Muscle Tenden Unit 2/Activation Dynamics1 ==
  data: u input; d_n_force_act output; act input; Tact input; Tdeact input
function d_n_force_act = d_n_force_act(u,act,Tact,Tdeact)
%#codegen    
%Rate of change of activation
%Equation is taken from Zajac (1989) Eq. 1
    B=Tact/Tdeact;
    d_n_force_act= u/Tact - (1/Tact*(B+(1-B)*u))*act;
end

== matlab function arm/Muscle Tenden Unit 2/Active Muscle Dynamics1 ==
  data: activation input; L0m input; Lm input; Vmax input; Vmus input; Fmax_mus input; muscle_force output
function muscle_force   =...
    muscle_dynamics(activation,L0m,Lm,Vmax,Vmus,Fmax_mus)
%#codegen

    %Hill Type Muscle F-V relationship.  Returns a normalized force-velocity value
    if (Vmus<Vmax)
        n_force_velocity=0;
    else
        if (Vmus >= Vmax && Vmus < 0)
            n_force_velocity = ((1-(Vmus/Vmax))/(1+(Vmus/0.17/Vmax)));
        else
            n_force_velocity =(1.8-0.8*((1+(Vmus/Vmax))/(1-7.56*Vmus/0.17/Vmax)));
        end
    end
    
    %Active muscle F-L relationships.  Returns a normalized F-L value

    a = 3.1108;
    b = .8698;
    s = .3914;

    if Lm < 0
        Lm = 0;
    end

    n_force_length = exp(-(abs(((Lm/L0m)^b-1)/s))^a);

    %Total active force of muscle based on normalized F-V and F-L relationships
    muscle_force = Fmax_mus* activation * n_force_velocity * n_force_length;
end

== matlab function arm/Muscle Tenden Unit 2/Metabolic Cost ==
  data: P_met output; act input; vmus input
function P_met = metabolic_cost(act, vmus)

    vmax = -0.45;
    Fmax = 6000;

    isLengthening = vmus > 0;
    isShortening = vmus <= 0; 

    psi = (0.01-(0.11*(vmus/vmax))+(0.06*exp(23*vmus/vmax))).*isLengthening;
    psi = psi + (0.23-0.16*exp(-8*vmus/vmax)).*isShortening;

    P_met = psi.*act.*abs(Fmax*vmax);

end

== matlab function arm/Muscle Tenden Unit 2/Passive Muscle dynamics1 ==
  data: pass_force output; L_m input; L0m input; fmax input
function pass_force = pmuscle_dynamics(L_m, L0m,fmax)
%#codegen
%passive CE F_L taken from Rubenson et. al.

%Passive muscle force
A = 2.38*10^(-2);
b = 5.31;

if L_m > 0    
    pass_force= fmax*A*exp(b*((L_m/L0m)-1));
else
    pass_force=0;
end


end

== matlab function arm/Muscle Tenden Unit 2/Tendon Dynamics1 ==
  data: kt input; L_t output; muscle_force input; Lt_slack input; fmax input
function L_t = L_tendon(kt,muscle_force,Lt_slack,fmax)
%#codegen
%Lichtwark, G.A. and Wilson, A.M., 2008. Journal of theoretical biology, 252(4), pp.662-673.
%Total tendon length
dL_t = (muscle_force + (fmax*log((-9*exp(-(20*muscle_force)/fmax)) + 10))/20)/kt;
L_t = dL_t + Lt_slack ;

end
